simulink model "ClosedLoopSystem"  (R2024b)
settings: Solver=FixedStepDiscrete  StartTime=0.0  StopTime=100  MaxStep=0.001  RelTol=1e-5
undefined symbols (not defined in the file or in its folder): DiscIntNeverNeededParam
libraries: slpidlib x1
settings Model: DataDictionary=eomParameters.sldd  Creator=nilgunozbulbul  LastModifiedBy=nilgunozbulbul
settings SolverCC: InitialStep=0.001

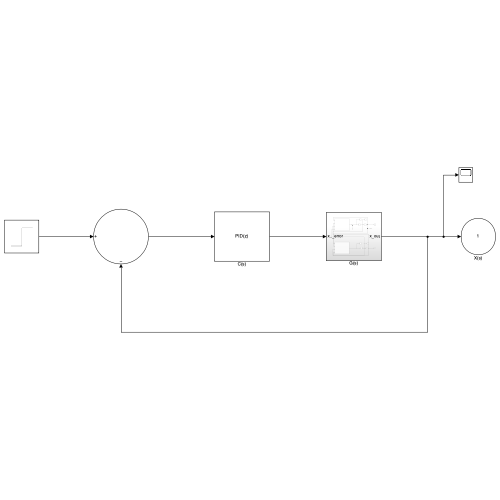
[thumbnail: Simulink's stored preview of the top-level diagram]
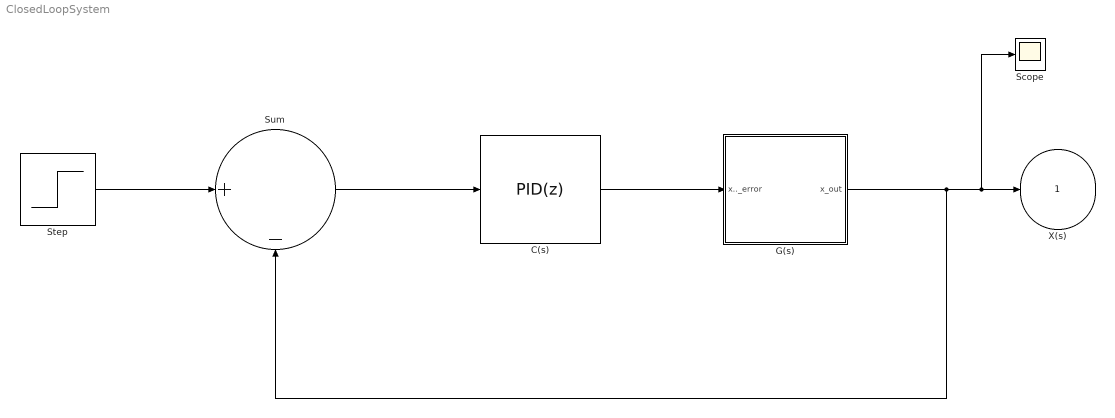
== system ClosedLoopSystem ==
  C(s) : slpidlib/PID Controller  Controller=PID  Form=Parallel  TimeDomain=Discrete-time  UseExternalTs=off  SampleTime=0.05  IntegratorMethod=Forward Euler  FilterMethod=Forward Euler  ControllerParametersSource=internal  P=0.2  I=0  UseKiTs=off  D=0  UseExternalDerivativeSource=off  N=100  UseFilter=on  TunerSelectOption=Transfer Function Based (PID Tuner App)  InitialConditionSource=internal  InitialConditionForIntegrator=0  InitialConditionForFilter=0  DifferentiatorICPrevScaledInput=0  ExternalReset=none  TrackingMode=off  Kt=1  LimitOutput=off  SatLimitsSource=internal  UpperSaturationLimit=inf  LowerSaturationLimit=-inf  LinearizeAsGain=off  AntiWindupMode=none  Kb=1  LimitIntegrator=off  UpperIntegratorSaturationLimit=inf  LowerIntegratorSaturationLimit=-inf  POutMin=[]  POutMax=[]  IOutMin=[]  IOutMax=[]  DOutMin=[]  DOutMax=[]  NOutMin=[]  NOutMax=[]  SumOutMin=[]  SumOutMax=[]  SaturationOutMin=[]  SaturationOutMax=[]  PParamMin=[]  PParamMax=[]  IParamMin=[]  IParamMax=[]  DParamMin=[]  DParamMax=[]  NParamMin=[]  NParamMax=[]  KbParamMin=[]  KbParamMax=[]  KtParamMin=[]  KtParamMax=[]  KbOutMin=[]  KbOutMax=[]  KtOutMin=[]  KtOutMax=[]  IntegratorOutMin=[]  IntegratorOutMax=[]  FilterOutMin=[]  FilterOutMax=[]  SumI1OutMin=[]  SumI1OutMax=[]  SumI2OutMin=[]  SumI2OutMax=[]  SumI3OutMin=[]  SumI3OutMax=[]  SumI4OutMin=[]  SumI4OutMax=[]  SumDOutMin=[]  SumDOutMax=[]  DifferentiatorOutMin=[]  DifferentiatorOutMax=[]  FilterDiffOutCoefMin=[]  FilterDiffOutCoefMax=[]  ReciprocalOutMin=[]  ReciprocalOutMax=[]  SumDenOutMin=[]  SumDenOutMax=[]  SumNumOutMin=[]  SumNumOutMax=[]  DivideOutMin=[]  DivideOutMax=[]  UdiffTsProdOutMin=[]  UdiffTsProdOutMax=[]  NTsProdOutMin=[]  NTsProdOutMax=[]  UintegralTsProdOutMin=[]  UintegralTsProdOutMax=[]  UngainTsProdOutMin=[]  UngainTsProdOutMax=[]  ClampingZeroOutDataTypeStr=Inherit: Inherit via back propagation  ClampingZeroOutMin=[]  ClampingZeroOutMax=[]  FilterDenConstantOutDataTypeStr=Inherit: Inherit via back propagation  FilterDenConstantOutMin=[]  FilterDenConstantOutMax=[]  PCopyOutDataTypeStr=Inherit: Inherit via back propagation  PCopyOutMin=[]  PCopyOutMax=[]  NCopyOutDataTypeStr=Inherit: Inherit via back propagation  NCopyOutMin=[]  NCopyOutMax=[]  IntegratorContinuousStateAttributes=''  IntegratorStateMustResolveToSignalObject=off  IntegratorRTWStateStorageClass=Auto  FilterContinuousStateAttributes=''  FilterStateMustResolveToSignalObject=off  FilterRTWStateStorageClass=Auto  ParallelPVariant=InternalParameters  IdealPVariant=Disabled  IVariant=InternalParameters  DVariant=InternalParameters  IntegratorVariant=Discrete  SatVariant=Disabled  AWVariant=Passthrough  PCopyVariant=Disabled  TRVariant=Disabled  FdbkBlocksVariant=Forward  IdealPFdbkVariant=Disabled  SatFdbkVariant=Disabled  DerivativeFilterVariant=ForwardEulerFilter  NVariant=InternalParameters  NCopyVariant=Disabled  FilterICVariant=InternalICsFilter  IntegratorICVariant=InternalICs  ExternalResetVariant=Disabled  TRSumVariant=Passthrough  SumFdbkVariant=Disabled  SumVariant=Sum_PID  TsampFilterVariant=InternalTs  TsampNgainVariant=Passthrough  TsampIntegralVariant=Disabled_SignalSpec  ExternalSaturationOutDataTypeStr=Inherit: Same as second input  DerivativeSourceVariant=ErrorSignal  PreIntVariant=InternalPreInt
      settings: LibrarySourceBlock=simulink/Discrete/Discrete PID Controller
  G(s) : Subsystem
  Scope : Scope
  Step : Step  Time=0  After=5  SampleTime=0.05
  Sum : Sum  Inputs=|+-
  X(s) : Outport
  wires:
  C(s)/1 -> G(s)/1(x.._error)
  Sum/1 -> C(s)/1
  G(s)/1(x_out) -> Scope/1, X(s)/1, Sum/2
  Step/1 -> Sum/1

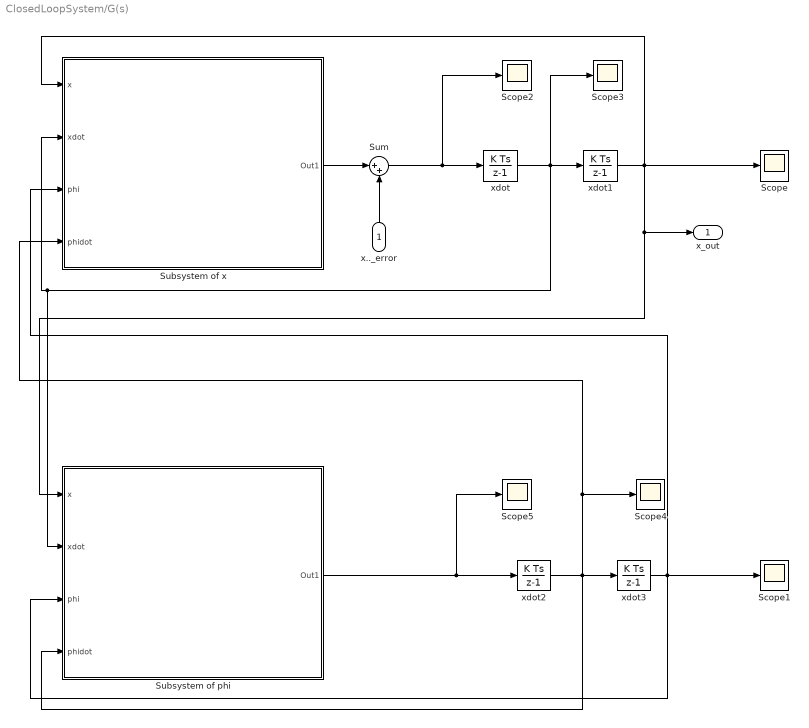
== system ClosedLoopSystem/G(s) ==
  x.._error : Inport
  Scope{,1..5} (6 alike) : Scope
  Subsystem of phi : Subsystem
  Subsystem of x : Subsystem
  Sum : Sum  Inputs=|++
  xdot{,1..3} (4 alike) : DiscreteIntegrator  SampleTime=0.05  ICPrevOutput=DiscIntNeverNeededParam  ICPrevScaledInput=DiscIntNeverNeededParam
  x_out : Outport
  wires:
  Subsystem of x/1(Out1) -> Sum/1
  x.._error/1 -> Sum/2
  Subsystem of phi/1(Out1) -> xdot2/1, Scope5/1
  xdot/1 -> xdot1/1, Scope3/1, Subsystem of phi/2(xdot), Subsystem of x/2(xdot)
  Sum/1 -> xdot/1, Scope2/1
  xdot1/1 -> x_out/1, Subsystem of phi/1(x), Subsystem of x/1(x), Scope/1
  xdot2/1 -> xdot3/1, Scope4/1, Subsystem of x/4(phidot), Subsystem of phi/4(phidot)
  xdot3/1 -> Scope1/1, Subsystem of x/3(phi), Subsystem of phi/3(phi)

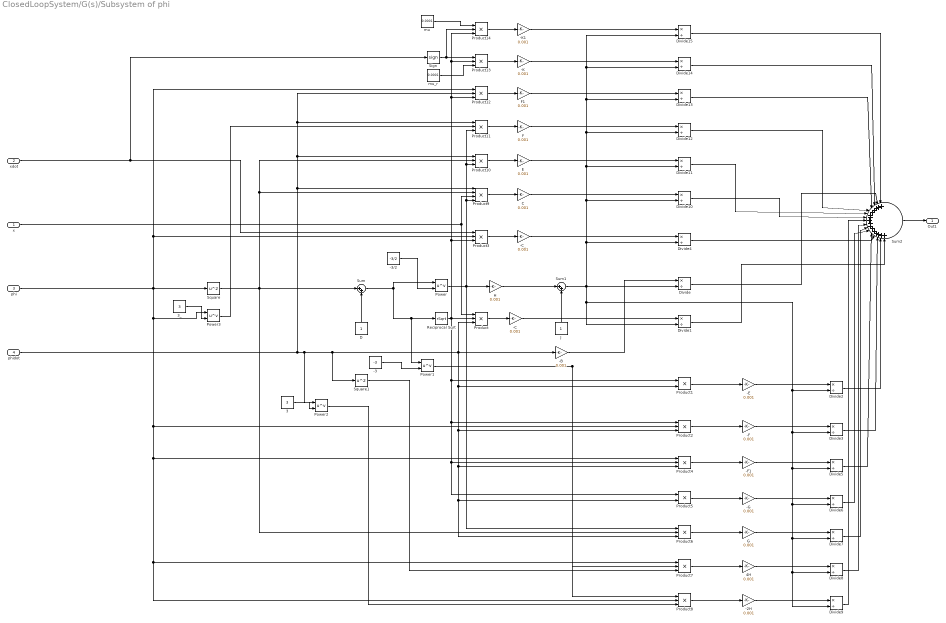
== system ClosedLoopSystem/G(s)/Subsystem of phi ==
  x : Inport
  xdot : Inport  Port=2
  phi : Inport  Port=3
  phidot : Inport  Port=4
  -2H : Gain  Gain=0.001
  -3 : Constant  Value=-3
  -3/2 : Constant  Value=-3/2
  -B : Gain  Gain=0.001
  -C : Gain  Gain=0.001
  -C_ : Gain  Gain=0.001
  -E : Gain  Gain=0.001
  -F : Gain  Gain=0.001
  -F1 : Gain  Gain=0.001
  -G : Gain  Gain=0.001
  -K : Gain  Gain=0.001
  -K1 : Gain  Gain=0.001
  3 : Constant  Value=3
  3_ : Constant  Value=3
  4H : Gain  Gain=0.001
  C : Gain  Gain=0.001
  D : Constant
  Divide{,1..15} (16 alike) : Product  Inputs=*/
  E : Gain  Gain=0.001
  F : Gain  Gain=0.001
  F1 : Gain  Gain=0.001
  G : Gain  Gain=0.001
  H : Gain  Gain=0.001
  J : Constant
  Power{,1..3} (4 alike) : Math  Operator=pow
  Product{,2..4,6..8,10..14} (12 alike) : Product  Inputs=3
  Product1 : Product
  Product5 : Product
  Product9 : Product  Inputs=4
  Reciprocal Sqrt : Sqrt  Operator=rSqrt
  Sign : Signum  ZeroCross=off
  Square : Math  Operator=square
  Square1 : Math  Operator=square
  Sum : Sum  Inputs=|++
  Sum1 : Sum  Inputs=|++
  Sum2 : Sum  Inputs=|++++++++++++++++
  mu : Constant  Value=0.0001
  mu_r : Constant  Value=0.0001
  Out1 : Outport
  wires:
  Square/1 -> Product10/2, Product9/2, Product6/2, Sum/1
  D/1 -> Sum/2
  Sum/1 -> Power1/1, Reciprocal Sqrt/1, Power/1
  Power/1 -> Product11/3, Product10/3, Product9/4, Product6/1, H/1
  H/1 -> Sum1/1
  J/1 -> Sum1/2
  phidot/1 -> Power2/1, Square1/1, Product6/3, Product5/2, Product4/3, Product2/3, Product1/2, Product/3, -B/1, Product12/2, Product11/1, Product10/1, Product9/1
  -B/1 -> Divide/1
  Sum1/1 -> Divide15/2, Divide14/2, Divide13/2, Divide12/2, Divide11/2, Divide10/2, Divide4/2, Divide9/2, Divide8/2, Divide7/2, Divide6/2, Divide5/2, Divide3/2, Divide2/2, Divide1/2, Divide/2
  Sum2/1 -> Out1/1
  x/1 -> Product/1, Product9/3
  Product/1 -> -C/1
  -C/1 -> Divide1/1
  Divide1/1 -> Sum2/16
  Product1/1 -> -E/1
  -E/1 -> Divide2/1
  Divide2/1 -> Sum2/15
  phi/1 -> Product12/1, Product3/2, Power3/1, Product8/2, Product7/1, Product4/1, Product2/2, Square/1
  Product2/1 -> -F/1
  -F/1 -> Divide3/1
  Divide3/1 -> Sum2/14
  xdot/1 -> Sign/1, Product3/1
  Product3/1 -> -C_/1
  -C_/1 -> Divide4/1
  Divide4/1 -> Sum2/13
  Reciprocal Sqrt/1 -> Product14/3, Product13/2, Product12/3, Product3/3, Product5/1, Product4/2, Product2/1, Product1/1, Product/2
  Product4/1 -> -F1/1
  -F1/1 -> Divide5/1
  Divide5/1 -> Sum2/12
  Product5/1 -> -G/1
  -G/1 -> Divide6/1
  Divide6/1 -> Sum2/11
  Product6/1 -> G/1
  G/1 -> Divide7/1
  Divide7/1 -> Sum2/10
  Square1/1 -> Product7/3
  Power1/1 -> Product8/1, Product7/2
  Product7/1 -> 4H/1
  4H/1 -> Divide8/1
  Divide8/1 -> Sum2/9
  Power2/1 -> Product8/3
  Product8/1 -> -2H/1
  -2H/1 -> Divide9/1
  Divide9/1 -> Sum2/8
  Product9/1 -> C/1
  C/1 -> Divide10/1
  Divide10/1 -> Sum2/7
  Product10/1 -> E/1
  E/1 -> Divide11/1
  Divide11/1 -> Sum2/6
  Power3/1 -> Product11/2
  Product11/1 -> F/1
  F/1 -> Divide12/1
  Divide12/1 -> Sum2/5
  Product12/1 -> F1/1
  F1/1 -> Divide13/1
  Divide13/1 -> Sum2/4
  Sign/1 -> Product14/2, Product13/1
  mu_r/1 -> Product13/3
  Product13/1 -> -K/1
  -K/1 -> Divide14/1
  Divide14/1 -> Sum2/3
  Divide/1 -> Sum2/2
  mu/1 -> Product14/1
  Product14/1 -> -K1/1
  -K1/1 -> Divide15/1
  Divide15/1 -> Sum2/1
  -3/2/1 -> Power/2
  -3/1 -> Power1/2
  3/1 -> Power2/2
  3_/1 -> Power3/2

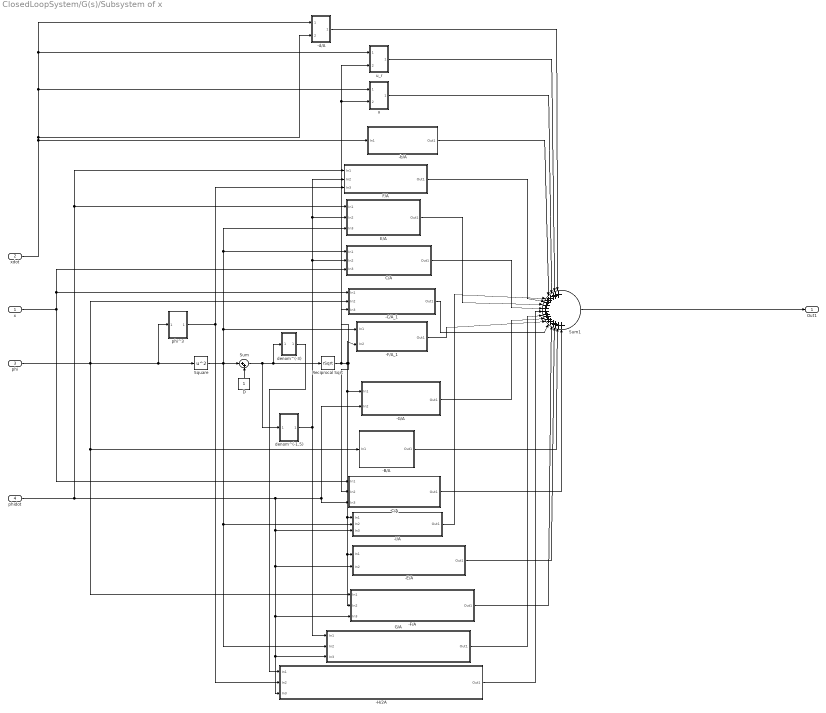
== system ClosedLoopSystem/G(s)/Subsystem of x ==
  x : Inport
  xdot : Inport  Port=2
  phi : Inport  Port=3
  phidot : Inport  Port=4
  -B/A : Subsystem
  -C/A : Subsystem
  -C/A_1 : Subsystem
  -E/A : Subsystem
  -F/A : Subsystem
  -F/A_1 : Subsystem
  -G/A : Subsystem
  -H/2A : Subsystem
  -I/A : Subsystem
  -b/A : Subsystem
  -d/A : Subsystem
  C/A : Subsystem
  D : Constant
  E/A : Subsystem
  F/A : Subsystem
  G/A : Subsystem
  Reciprocal Sqrt : Sqrt  Operator=rSqrt
  Square : Math  Operator=square
  Sum : Sum  Inputs=|++
  Sum1 : Sum  Inputs=|+++++++++++++++++
  denom^(-1.5) : Subsystem
  denom^(-3) : Subsystem
  phi^3 : Subsystem
  u : Subsystem
  u_r : Subsystem
  Out1 : Outport
  wires:
  phi/1 -> -C/A_1/2(In2), -F/A/1(In1), -B/A/1(In1), Square/1, phi^3/1(In1)
  Square/1 -> G/A/2(In2), -I/A/2(In2), -F/A_1/1(In1), E/A/3(In3), C/A/1(In1), Sum/1
  D/1 -> Sum/2
  Sum1/1 -> Out1/1
  phidot/1 -> F/A/1(In1), E/A/1(In1), -I/A/3(In3), -E/A/2(In2), -F/A/3(In3), G/A/3(In3), -H/2A/3(In3), -G/A/2(In2), -C/A/3(In3)
  Reciprocal Sqrt/1 -> u_r/2(In2), u/2(In2), -F/A_1/2(In2), -F/A/2(In2), -E/A/1(In1), -I/A/1(In1), -G/A/1(In1), -C/A_1/3(In3), -C/A/2(In2)
  x/1 -> -C/A/1(In1), C/A/3(In3), -C/A_1/1(In1)
  xdot/1 -> -d/A/2(In2), u/1(In1), -d/A/1(In1), u_r/1(In1), -b/A/1(In1)
  Sum/1 -> Reciprocal Sqrt/1, denom^(-3)/1(In1), denom^(-1.5)/1(In1)
  -H/2A/1(Out1) -> Sum1/9
  G/A/1(Out1) -> Sum1/10
  -F/A/1(Out1) -> Sum1/14
  -E/A/1(Out1) -> Sum1/15
  -I/A/1(Out1) -> Sum1/5
  -C/A/1(Out1) -> Sum1/17
  -B/A/1(Out1) -> Sum1/16
  -G/A/1(Out1) -> Sum1/11
  -F/A_1/1(Out1) -> Sum1/12
  -C/A_1/1(Out1) -> Sum1/13
  C/A/1(Out1) -> Sum1/8
  E/A/1(Out1) -> Sum1/7
  F/A/1(Out1) -> Sum1/6
  -b/A/1(Out1) -> Sum1/4
  u/1(Out1) -> Sum1/3
  u_r/1(Out1) -> Sum1/2
  -d/A/1(Out1) -> Sum1/1
  phi^3/1(Out1) -> -H/2A/2(In2), F/A/3(In3)
  denom^(-1.5)/1(Out1) -> C/A/2(In2), F/A/2(In2), E/A/2(In2), G/A/1(In1)
  denom^(-3)/1(Out1) -> -H/2A/1(In1)

== system ClosedLoopSystem/G(s)/Subsystem of x/-B//A ==
  In1 : Inport
  -B/A : Gain  Gain=0.001
  Out1 : Outport
  wires:
  In1/1 -> -B/A/1
  -B/A/1 -> Out1/1

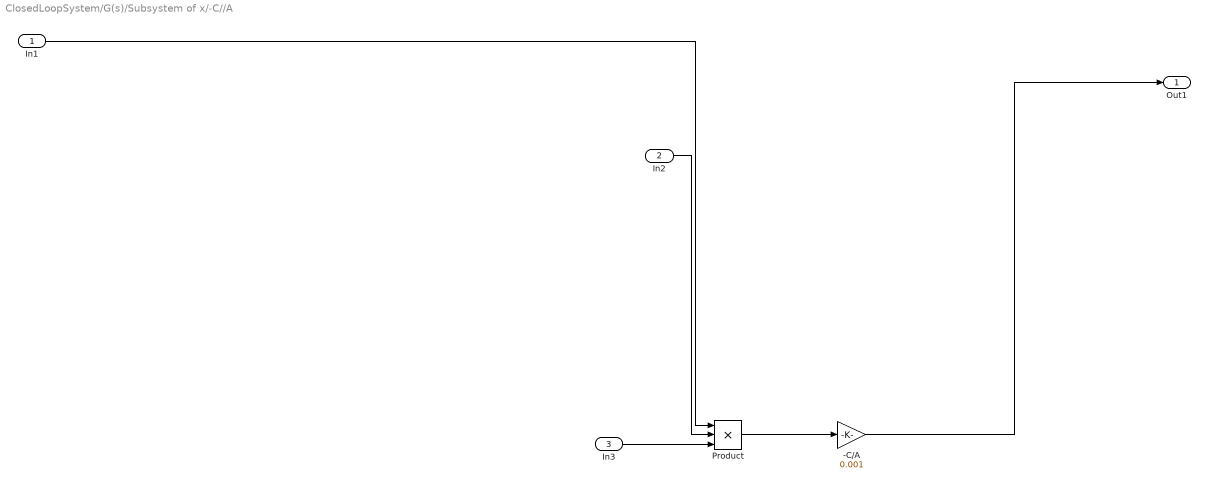
== system ClosedLoopSystem/G(s)/Subsystem of x/-C//A ==
  In1 : Inport
  In2 : Inport  Port=2
  In3 : Inport  Port=3
  -C/A : Gain  Gain=0.001
  Product : Product  Inputs=3
  Out1 : Outport
  wires:
  In3/1 -> Product/3
  In1/1 -> Product/1
  In2/1 -> Product/2
  -C/A/1 -> Out1/1
  Product/1 -> -C/A/1

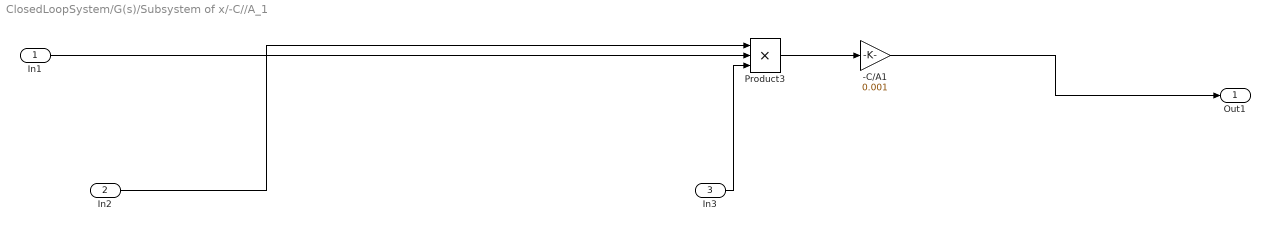
== system ClosedLoopSystem/G(s)/Subsystem of x/-C//A_1 ==
  In1 : Inport
  In2 : Inport  Port=2
  In3 : Inport  Port=3
  -C/A1 : Gain  Gain=0.001
  Product3 : Product  Inputs=3
  Out1 : Outport
  wires:
  In1/1 -> Product3/2
  In3/1 -> Product3/3
  -C/A1/1 -> Out1/1
  In2/1 -> Product3/1
  Product3/1 -> -C/A1/1

== system ClosedLoopSystem/G(s)/Subsystem of x/-E//A ==
  In1 : Inport
  In2 : Inport  Port=2
  -E/A : Gain  Gain=0.001
  Product1 : Product
  Out1 : Outport
  wires:
  In2/1 -> Product1/2
  -E/A/1 -> Out1/1
  In1/1 -> Product1/1
  Product1/1 -> -E/A/1

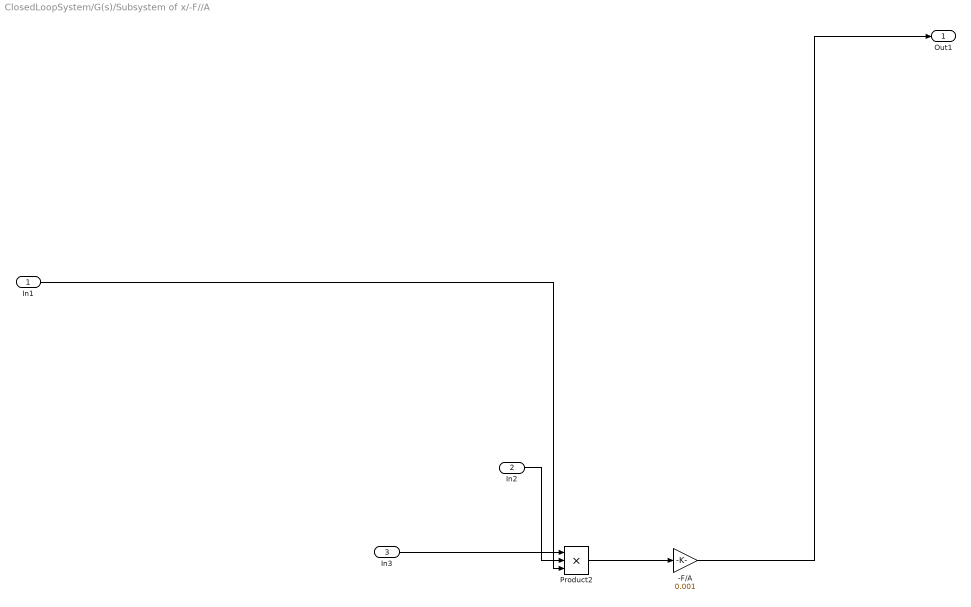
== system ClosedLoopSystem/G(s)/Subsystem of x/-F//A ==
  In1 : Inport
  In2 : Inport  Port=2
  In3 : Inport  Port=3
  -F/A : Gain  Gain=0.001
  Product2 : Product  Inputs=3
  Out1 : Outport
  wires:
  -F/A/1 -> Out1/1
  In2/1 -> Product2/2
  In3/1 -> Product2/1
  In1/1 -> Product2/3
  Product2/1 -> -F/A/1

== system ClosedLoopSystem/G(s)/Subsystem of x/-F//A_1 ==
  In1 : Inport
  In2 : Inport  Port=2
  -F/A2 : Gain  Gain=0.001
  Product4 : Product
  Out1 : Outport
  wires:
  -F/A2/1 -> Out1/1
  In1/1 -> Product4/2
  In2/1 -> Product4/1
  Product4/1 -> -F/A2/1

== system ClosedLoopSystem/G(s)/Subsystem of x/-G//A ==
  In1 : Inport
  In2 : Inport  Port=2
  -G/A : Gain  Gain=0.001
  Product5 : Product
  Out1 : Outport
  wires:
  In2/1 -> Product5/2
  -G/A/1 -> Out1/1
  In1/1 -> Product5/1
  Product5/1 -> -G/A/1

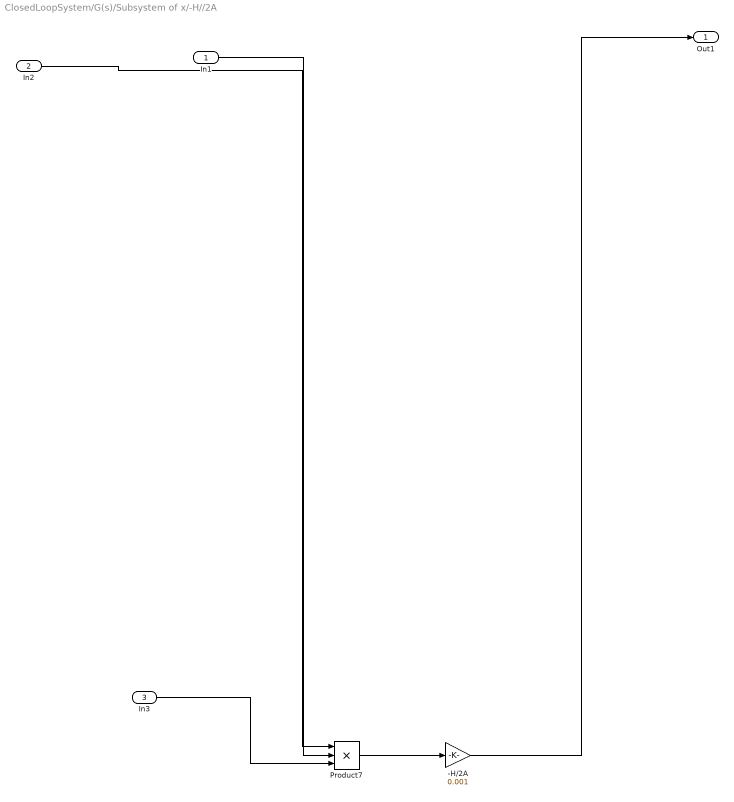
== system ClosedLoopSystem/G(s)/Subsystem of x/-H//2A ==
  In1 : Inport
  In2 : Inport  Port=2
  In3 : Inport  Port=3
  -H/2A : Gain  Gain=0.001
  Product7 : Product  Inputs=3
  Out1 : Outport
  wires:
  In2/1 -> Product7/1
  In1/1 -> Product7/2
  In3/1 -> Product7/3
  -H/2A/1 -> Out1/1
  Product7/1 -> -H/2A/1

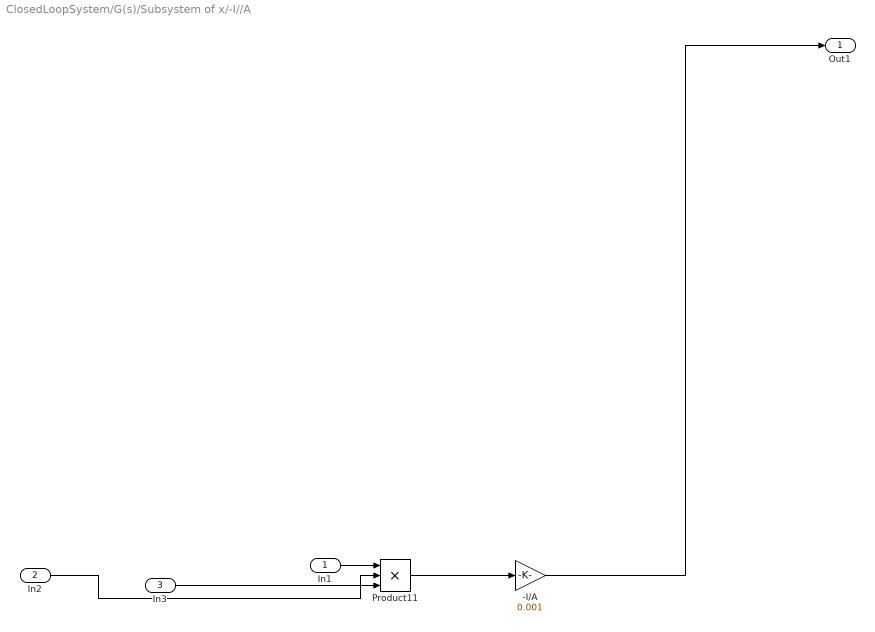
== system ClosedLoopSystem/G(s)/Subsystem of x/-I//A ==
  In1 : Inport
  In2 : Inport  Port=2
  In3 : Inport  Port=3
  -I/A : Gain  Gain=0.001
  Product11 : Product  Inputs=3
  Out1 : Outport
  wires:
  -I/A/1 -> Out1/1
  In3/1 -> Product11/3
  In2/1 -> Product11/2
  In1/1 -> Product11/1
  Product11/1 -> -I/A/1

== system ClosedLoopSystem/G(s)/Subsystem of x/-b//A ==
  In1 : Inport
  -b/A : Gain  Gain=0.001
  Out1 : Outport
  wires:
  In1/1 -> -b/A/1
  -b/A/1 -> Out1/1

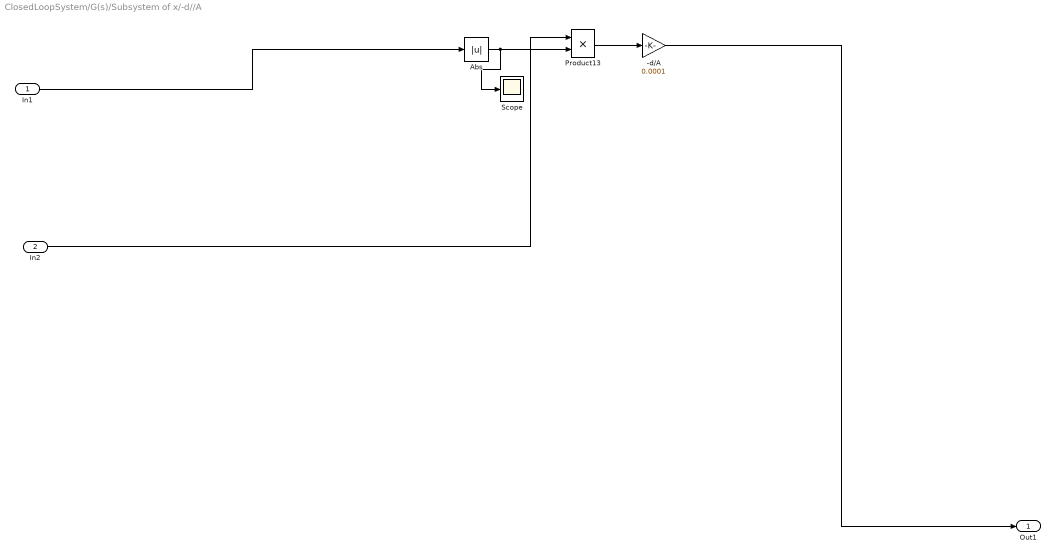
== system ClosedLoopSystem/G(s)/Subsystem of x/-d//A ==
  In1 : Inport
  In2 : Inport  Port=2
  -d/A : Gain  Gain=0.0001
  Abs : Abs  ZeroCross=off  SaturateOnIntegerOverflow=off
  Product13 : Product
  Scope : Scope
  Out1 : Outport
  wires:
  Product13/1 -> -d/A/1
  In1/1 -> Abs/1
  In2/1 -> Product13/1
  -d/A/1 -> Out1/1
  Abs/1 -> Scope/1, Product13/2

== system ClosedLoopSystem/G(s)/Subsystem of x/C//A ==
  In1 : Inport
  In2 : Inport  Port=2
  In3 : Inport  Port=3
  C/A : Gain  Gain=0.001
  Product8 : Product  Inputs=3
  Out1 : Outport
  wires:
  C/A/1 -> Out1/1
  In2/1 -> Product8/3
  In3/1 -> Product8/1
  In1/1 -> Product8/2
  Product8/1 -> C/A/1

== system ClosedLoopSystem/G(s)/Subsystem of x/E//A ==
  In1 : Inport
  In2 : Inport  Port=2
  In3 : Inport  Port=3
  E/A : Gain  Gain=0.001
  Product9 : Product  Inputs=3
  Out1 : Outport
  wires:
  E/A/1 -> Out1/1
  In2/1 -> Product9/3
  In1/1 -> Product9/1
  In3/1 -> Product9/2
  Product9/1 -> E/A/1

== system ClosedLoopSystem/G(s)/Subsystem of x/F//A ==
  In1 : Inport
  In2 : Inport  Port=2
  In3 : Inport  Port=3
  F/A : Gain  Gain=0.0001
  Product10 : Product  Inputs=3
  Out1 : Outport
  wires:
  In3/1 -> Product10/2
  F/A/1 -> Out1/1
  In2/1 -> Product10/3
  In1/1 -> Product10/1
  Product10/1 -> F/A/1

== system ClosedLoopSystem/G(s)/Subsystem of x/G//A ==
  In1 : Inport
  In2 : Inport  Port=2
  In3 : Inport  Port=3
  G/A : Gain  Gain=0.001
  Product6 : Product  Inputs=3
  Out1 : Outport
  wires:
  G/A/1 -> Out1/1
  In1/1 -> Product6/2
  In3/1 -> Product6/3
  In2/1 -> Product6/1
  Product6/1 -> G/A/1

== system ClosedLoopSystem/G(s)/Subsystem of x/denom^(-1.5) ==
  In1 : Inport
  3/2 : Constant  Value=-1.5
  Power1 : Math  Operator=pow
  Out1 : Outport
  wires:
  In1/1 -> Power1/1
  Power1/1 -> Out1/1
  3/2/1 -> Power1/2

== system ClosedLoopSystem/G(s)/Subsystem of x/denom^(-3) ==
  In1 : Inport
  3 : Constant  Value=-3
  Power2 : Math  Operator=pow
  Out1 : Outport
  wires:
  Power2/1 -> Out1/1
  In1/1 -> Power2/1
  3/1 -> Power2/2

== system ClosedLoopSystem/G(s)/Subsystem of x/phi^3 ==
  In1 : Inport
  3_ : Constant  Value=3
  Power3 : Math  Operator=pow
  Out1 : Outport
  wires:
  Power3/1 -> Out1/1
  In1/1 -> Power3/1
  3_/1 -> Power3/2

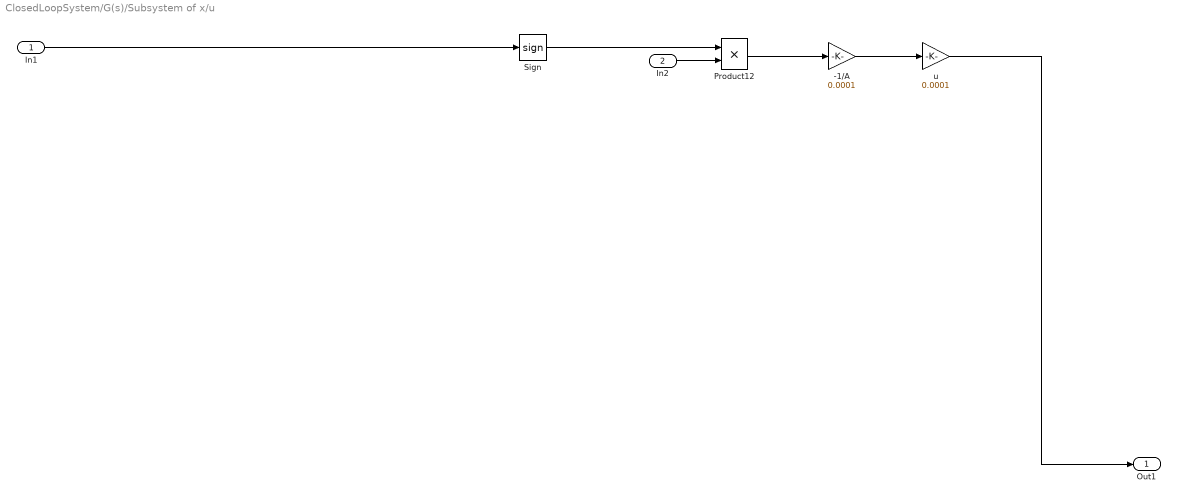
== system ClosedLoopSystem/G(s)/Subsystem of x/u ==
  In1 : Inport
  In2 : Inport  Port=2
  -1/A : Gain  Gain=0.0001
  Product12 : Product
  Sign : Signum  ZeroCross=off
  u : Gain  Gain=0.0001
  Out1 : Outport
  wires:
  In2/1 -> Product12/2
  Sign/1 -> Product12/1
  In1/1 -> Sign/1
  u/1 -> Out1/1
  Product12/1 -> -1/A/1
  -1/A/1 -> u/1

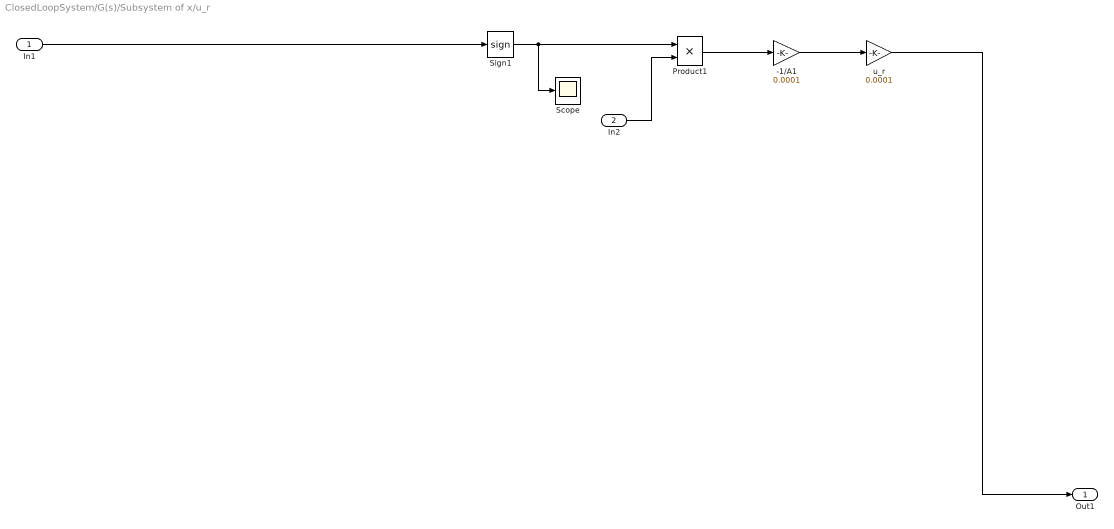
== system ClosedLoopSystem/G(s)/Subsystem of x/u_r ==
  In1 : Inport
  In2 : Inport  Port=2
  -1/A1 : Gain  Gain=0.0001
  Product1 : Product
  Scope : Scope
  Sign1 : Signum  ZeroCross=off
  u_r : Gain  Gain=0.0001
  Out1 : Outport
  wires:
  Product1/1 -> -1/A1/1
  -1/A1/1 -> u_r/1
  Sign1/1 -> Scope/1, Product1/1
  In1/1 -> Sign1/1
  In2/1 -> Product1/2
  u_r/1 -> Out1/1
